simulink subsystem "Encoder_SubSystem"  (R2020b)
settings: Solver=VariableStepAuto  StartTime=0.0  StopTime=10.0  RelTol=1e-3
values from neighbouring files (symbols this model uses):
  n = gbox.N    [Electromechanical.m]
  Ts = 1e-2    (= 0.01)    [balrob_params.m]
undefined symbols (not defined in the file or in its folder): sens
settings Model: Creator=umberto  LastModifiedBy=umberto

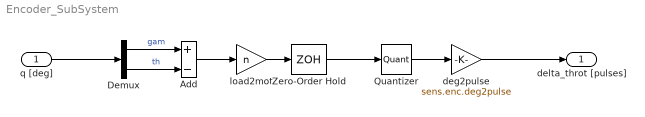
== system Encoder_SubSystem ==
  q [deg] : Inport
  Add : Sum  Inputs=+-
  Demux : Demux  Outputs=2
  Quantizer : Quantizer  QuantizationInterval=sens.enc.pulse2deg
  Zero-Order Hold : ZeroOrderHold  SampleTime=Ts
  deg2pulse : Gain  Gain=sens.enc.deg2pulse
  load2mot : Gain  Gain=n
  delta_throt [pulses] : Outport
  wires:
  deg2pulse/1 -> delta_throt [pulses]/1
  Quantizer/1 -> deg2pulse/1
  Zero-Order Hold/1 -> Quantizer/1
  load2mot/1 -> Zero-Order Hold/1
  Add/1 -> load2mot/1
  Demux/2 -> Add/2  "th"
  Demux/1 -> Add/1  "gam"
  q [deg]/1 -> Demux/1
